simulink subsystem "PipingAccumulatorSubsystem"  (R2026a)
settings: Solver=VariableStepAuto
undefined symbols (not defined in the file): accumulatorGasK, accumulatorInitVolumeL, accumulatorMinGasVolume, accumulatorPreChargeP, accumulatorStopD, accumulatorStopK, accumulatorTotalVolume, flowResistanceDpNom, flowResistanceMdotNom, pipingAddLength, pipingArea, pipingD, pipingLength, pipingRoughness, pLoop, TCoolantIn
libraries: fl_lib x3, SimscapeFluids_lib x2
settings Model: Creator=epelster  LastModifiedBy=epelster

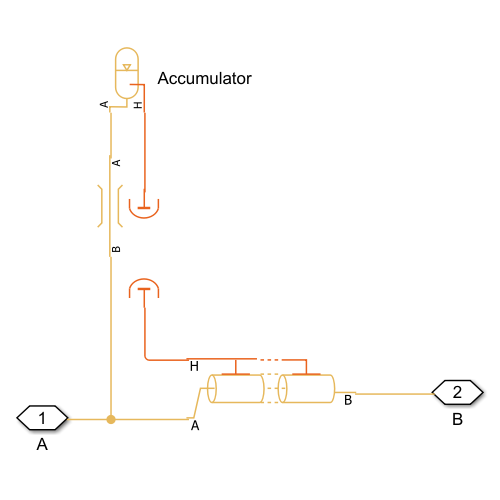
[thumbnail: Simulink's stored preview of the top-level diagram]
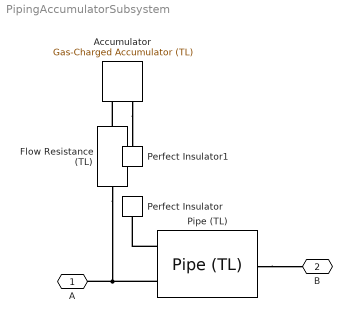
== system PipingAccumulatorSubsystem ==
  Accumulator : SimscapeFluids_lib/Thermal Liquid/Tanks & Accumulators/Gas-Charged Accumulator (TL)  capacity="accumulatorTotalVolume.value(\"l\") l"  dead_volume="accumulatorMinGasVolume.value(\"l\") l"  p_precharge_gauge="accumulatorPreChargeP.value(\"bar\") bar"  k_sh="accumulatorGasK.value(\"1\")"  area=pipingArea.value('mm^2') mm^2  stiff_coeff="accumulatorStopK.value(\"MPa/m^3\") MPa/m^3"  damping_coeff="accumulatorStopD.value(\"MPa*s/m^6\") MPa*s/m^6"  liquid_volume_specify=on  liquid_volume_priority=High  liquid_volume="accumulatorInitVolumeL.value(\"l\") l"  liquid_volume_nominal_specify=off  liquid_volume_nominal_value=1  liquid_volume_nominal_unit=m^3  liquid_mass_specify=off  liquid_mass_priority=None  liquid_mass=5 kg  liquid_mass_nominal_specify=off  liquid_mass_nominal_value=1  liquid_mass_nominal_unit=kg  p_I_specify=on  p_I_priority=High  p_I="pLoop.value(\"bar\") bar"  p_I_nominal_specify=off  p_I_nominal_value=1  p_I_nominal_unit=MPa  T_I_specify=on  T_I_priority=High  T_I=TCoolantIn.value('degC') degC  T_I_nominal_specify=off  T_I_nominal_value=1  T_I_nominal_unit=K
  Flow Resistance (TL) : fl_lib/Thermal Liquid/Elements/Flow Resistance (TL)  delta_p_nominal="flowResistanceDpNom.value(\"MPa\") MPa"  mdot_nominal="flowResistanceMdotNom.value(\"kg/s\") kg/s"  area=pipingArea.value('mm^2') mm^2  laminar_fraction=1e-3
  Perfect Insulator : fl_lib/Thermal/Thermal Elements/Perfect Insulator  T_specify=off  T_priority=None  T=293.15 K  T_nominal_specify=off  T_nominal_value=1  T_nominal_unit=K
  Perfect Insulator1 : fl_lib/Thermal/Thermal Elements/Perfect Insulator  T_specify=off  T_priority=None  T=293.15 K  T_nominal_specify=off  T_nominal_value=1  T_nominal_unit=K
  Pipe (TL) : SimscapeFluids_lib/Thermal Liquid/Pipes & Fittings/Pipe (TL)  dynamic_compressibility=true  inertia=false  num_segments=1  pipe_length=pipingLength.value('m') m  cross_section_geometry=fluids.thermal_liquid.pipes_fittings.enum.CrossSectionGeometry.Circular  pipe_diameter=pipingD.value('m') m  pipe_inner_diameter=0.05 m  pipe_outer_diameter=0.1 m  pipe_width=0.1 m  pipe_height=0.1 m  pipe_major_axis=0.1 m  pipe_minor_axis=0.05 m  pipe_side=0.1 m  pipe_angle=30 deg  area=0.01 m^2  Dh=0.1128 m  elevation_spec=foundation.enum.constant_variable.constant  elevation_gain=0 m  gravity_spec=foundation.enum.constant_variable.constant  g=9.81 m/s^2  pressure_loss_spec=fluids.thermal_liquid.pipes_fittings.enum.PressureLossSpec.Haaland  local_pressure_loss_spec=fluids.thermal_liquid.pipes_fittings.enum.LocalLossSpec.AggregateLength  length_add=pipingAddLength.value('m') m  loss_coefficient=0.1  roughness_spec=fluids.thermal_liquid.pipes_fittings.enum.RoughnessSpec.Custom  roughness=pipingRoughness.value('m') m  Re_friction_TLU=[400, 1000, 1500, 3000, 4000, 6000, 10000, 20000, 40000, 60000, 100000, 100000000]  friction_factor_TLU=[.264, .112, .071, .0417, .0387, .0268, .025, .0232, .0226, .022, .0214, .0214]  Re_lam=2000  Re_tur=4000  shape_factor=64  mdot_nominal=[.1, 1] kg/s  p_diff_nominal=[.001, .01] MPa  mdot_threshold=1e-6 kg/s  wall_spec=fluids.thermal_liquid.pipes_fittings.enum.wall_spec.rigid  vol_expansion_spec=fluids.thermal_liquid.pipes_fittings.enum.VolumeExpansionSpec.Area  area_pressure_gain=1e-6 m^2/MPa  static_pressure_TLU=[.1, 1] MPa  area_pressure_gain_TLU=[1e-05, 1.1e-05] m^2  material_behavior_spec=fluids.thermal_liquid.pipes_fittings.enum.PipeMaterialBehavior.Linear  diameter_pressure_gain=1e-6 m/MPa  wall_thickness=0.05 m  elastic_modulus=69 GPa  stress_TLU=[276, 310] MPa  strain_TLU=[.004, .02]  stress_assert_action=simscape.enum.assert.action.none  stress_max=400 MPa  poisson_ratio=0.33  wall_time_constant=0.01 s  thermal_expansion=false  alpha_L_wall=24 um/(deltaK*m)  thermal_expansion_Tref=293.15 K  heat_transfer_spec=fluids.thermal_liquid.pipes_fittings.enum.HeatTransferSpec.Gnielinski  mdot_nominal_heat=[.1, 1] kg/s  T_in_nominal=[293.15, 293.15] K  T_out_nominal=[300, 300] K  p_in_nominal_heat=[.101325, .101325] MPa  T_wall_nominal=[303.15, 303.15] K  a_coeff=0.023  b_Re_power=0.8  c_Pr_power=0.4  Nu_lam=3.66  Re_Colburn_TLU=[100, 150, 1000]  Colburn_factor_TLU=[.019, .013, .002]  Re_Nu_TLU=[100, 150, 1000]  Pr_Nu_TLU=[1, 10]  Nu_TLU=[3.72, 4.21; 3.75, 4.44; 4.21, 7.15]  p0_vec=pLoop.value('bar') bar  T0_vec=TCoolantIn.value('degC') degC  mdot0=0.1 kg/s  p_nominal=0.101325 MPa  T_nominal=293.15 K
  A : PMIOPort  Side=Left
  B : PMIOPort  Port=2  Side=Right
  connections:
  Flow Resistance (TL)/RConn1 -- Pipe (TL)/LConn1 -- A/RConn1
  Pipe (TL)/LConn2 -- Perfect Insulator/LConn1
  Accumulator/RConn2 -- Perfect Insulator1/LConn1
  Pipe (TL)/RConn1 -- B/RConn1
  Flow Resistance (TL)/LConn1 -- Accumulator/RConn1
